simulink model "SS_MIMO_DU_Restricciones_Simulink_P3"  (R2020b)
settings: Solver=ode45  StartTime=0.0  StopTime=30  RelTol=1e-3
InitFcn:
  | J1=0.001;
  | B1=0.05;
  | Km1=1;
  | 
  | J2=0.002;
  | B2=0.03;
  | Km2=1;
  | Kl=10;
values from neighbouring files (symbols this model uses):
  Td = 0.25    [Initialization_MPC_SS.m]
undefined symbols (not defined in the file or in its folder): nu, ny
settings Model: Creator=asierzubizarreta  LastModifiedBy=snopv
settings DataIOCC: LimitDataPoints=on  SaveFormat=Array  ReturnWorkspaceOutputs=off
settings OptimizationCC: BlockReduction=off  BooleanDataType=off  LifeSpan=inf
settings DebuggingCC: SaveWithParameterizedLinksMsg=none  UnderspecifiedInitializationDetection=Classic  MergeDetectMultiDrivingBlocksExec=none  SignalResolutionControl=TryResolveAllWithWarning  SFUnexpectedBacktrackingDiag=warning  SFNoUnconditionalDefaultTransitionDiag=warning  SFExecutionAtInitializationDiag=none  ArithmeticOperatorsInVariantConditions=warning
settings HardwareCC: ProdBitPerPointer=32  ProdBitPerSizeT=32  ProdBitPerPtrDiffT=32  ProdLargestAtomicFloat=None  ProdIntDivRoundTo=Undefined  ProdEndianess=Unspecified  ProdWordSize=32  ProdHWDeviceType=32-bit Generic  TargetUnknown=on
settings ModelReferenceCC: PropagateSignalLabelsOutOfModel=off
settings SFSimCC: SimUseLocalCustomCode=off  CustomCodeUndefinedFunction=UseInterfaceOnly
settings RTWCC: RTWUseLocalCustomCode=off
settings CodeAppCC: StateflowObjectComments=on
settings GRTTargetCC: TargetLangStandard=C89/C90 (ANSI)
settings ConfigComp: CovMetricSettings=dw  CovSaveCumulativeToWorkspaceVar=on  CovSaveSingleToWorkspaceVar=on  CovExternalEMLEnable=off  CovSFcnEnable=off

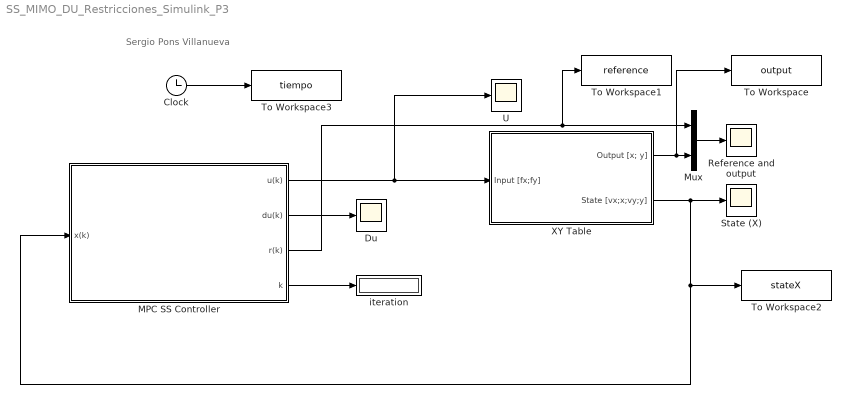
== system SS_MIMO_DU_Restricciones_Simulink_P3 ==
  note: Sergio Pons Villanueva
  Clock : Clock
  Du : Scope
  MPC SS Controller : Subsystem  InitFcn=|  TreatAsAtomicUnit=on
      | [parameters, Ref,Td]=Initialization_MPC_SS; 
      | [nx,nu]=size(parameters.B);
      | [ny,nx]=size(parameters.C);
      mask DialogControl DescGroupVar Prompt: MPC Controller
      mask Display:
      | fprintf('MPC SS Control\n\n\n');
      | 
      | 
      | port_label('output',1,'u(k)');
      | port_label('output',2,'du(k)');
      | port_label('output',3,'r(k)');
      | port_label('output',4,'k');
      | port_label('input',1,'x(k)');
  Mux : Mux  Inputs=2
  Reference and output : Scope
  State (X) : Scope
  To Workspace : ToWorkspace  VariableName=output  SaveFormat=Timeseries  SampleTime=-1
  To Workspace1 : ToWorkspace  VariableName=reference  SaveFormat=Timeseries  SampleTime=-1
  To Workspace2 : ToWorkspace  VariableName=stateX  SaveFormat=Timeseries  SampleTime=-1
  To Workspace3 : ToWorkspace  VariableName=tiempo  SaveFormat=Timeseries  SampleTime=-1
  U : Scope
  XY Table : Subsystem  SystemSampleTime=Td  mask{m1=0.5, m2=0.1, b1=0.5, b2=0.1, K1=0.01, K2=0.01}
      mask prompts: m1 "Mass 1"; m2 "Mass 2"; b1 "Friction (B1)"; b2 "Friction (B2)"; K1 "Coupling Constant (K1)"; K2 "Coupling Constant (K2)"
  iteration : Display
  wires:
  Mux/1 -> Reference and output/1
  XY Table/1(Output [x; y]) -> To Workspace/1, Mux/2
  MPC SS Controller/1(u(k)) -> U/1, XY Table/1(Input [fx;fy])
  MPC SS Controller/4(k) -> iteration/1
  MPC SS Controller/2(du(k)) -> Du/1
  MPC SS Controller/3(r(k)) -> To Workspace1/1, Mux/1
  XY Table/2(State [vx;x;vy;y]) -> MPC SS Controller/1(x(k)), To Workspace2/1, State (X)/1
  Clock/1 -> To Workspace3/1

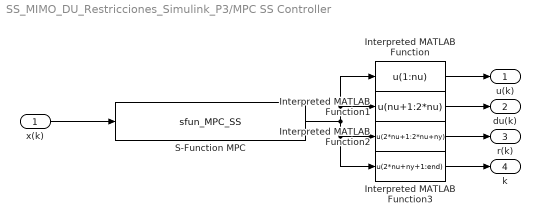
== system SS_MIMO_DU_Restricciones_Simulink_P3/MPC SS Controller ==
  x(k) : Inport
  Interpreted MATLAB Function : MATLABFcn  MATLABFcn=u(1:nu)
  Interpreted MATLAB Function1 : MATLABFcn  MATLABFcn=u(nu+1:2*nu)
  Interpreted MATLAB Function2 : MATLABFcn  MATLABFcn=u(2*nu+1:2*nu+ny)
  Interpreted MATLAB Function3 : MATLABFcn  MATLABFcn=u(2*nu+ny+1:end)
  S-Function MPC : S-Function  FunctionName=sfun_MPC_SS  SFunctionModules=s  SFunctionDeploymentMode=off  EnableBusSupport=off
  u(k) : Outport
  du(k) : Outport  Port=2
  r(k) : Outport  Port=3
  k : Outport  Port=4
  wires:
  Interpreted MATLAB Function/1 -> u(k)/1
  Interpreted MATLAB Function1/1 -> du(k)/1
  Interpreted MATLAB Function2/1 -> r(k)/1
  Interpreted MATLAB Function3/1 -> k/1
  x(k)/1 -> S-Function MPC/1
  S-Function MPC/1 -> Interpreted MATLAB Function1/1, Interpreted MATLAB Function/1, Interpreted MATLAB Function3/1, Interpreted MATLAB Function2/1

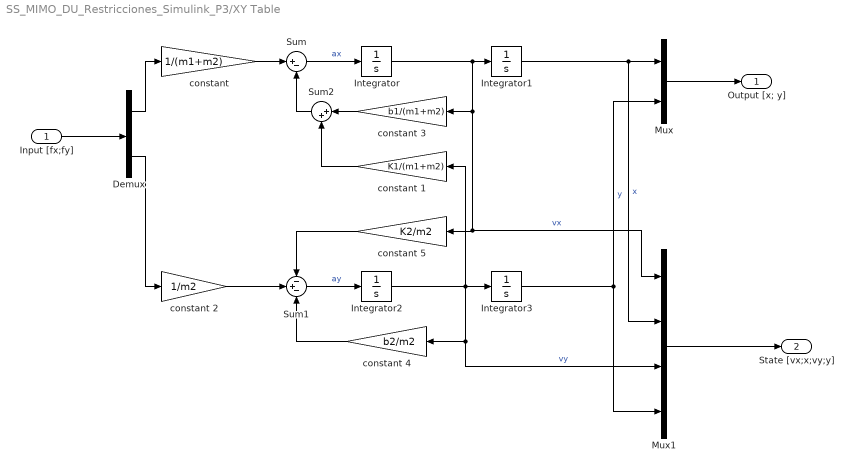
== system SS_MIMO_DU_Restricciones_Simulink_P3/XY Table ==
  Input [fx;fy] : Inport
  Demux : Demux  Outputs=2
  Integrator{,1..3} (4 alike) : Integrator
  Mux : Mux  Inputs=2
  Mux1 : Mux
  Sum : Sum  Inputs=|+-
  Sum1 : Sum  Inputs=-+-
  Sum2 : Sum  Inputs=|++
  constant : Gain  Gain=1/(m1+m2)
  constant 1 : Gain  Gain=K1/(m1+m2)
  constant 2 : Gain  Gain=1/m2
  constant 3 : Gain  Gain=b1/(m1+m2)
  constant 4 : Gain  Gain=b2/m2
  constant 5 : Gain  Gain=K2/m2
  Output [x; y] : Outport
  State [vx;x;vy;y] : Outport  Port=2
  wires:
  constant 4/1 -> Sum1/3
  Integrator1/1 -> Mux1/2, Mux/1  "x"
  Integrator/1 -> Mux1/1, constant 5/1, constant 3/1, Integrator1/1  "vx"
  Sum/1 -> Integrator/1  "ax"
  Integrator2/1 -> constant 1/1, Integrator3/1, constant 4/1, Mux1/3  "vy"
  Sum1/1 -> Integrator2/1  "ay"
  Mux/1 -> Output [x; y]/1
  Demux/1 -> constant/1
  Demux/2 -> constant 2/1
  Input [fx;fy]/1 -> Demux/1
  Mux1/1 -> State [vx;x;vy;y]/1
  constant 2/1 -> Sum1/2
  constant/1 -> Sum/1
  Integrator3/1 -> Mux/2, Mux1/4  "y"
  constant 3/1 -> Sum2/1
  Sum2/1 -> Sum/2
  constant 1/1 -> Sum2/2
  constant 5/1 -> Sum1/1
